simulink model "week14"  (R2018a)
settings: Solver=VariableStepAuto  StartTime=0.0  StopTime=15  RelTol=1e-3
values from neighbouring files (symbols this model uses):
  km = 0.5    [Parameters.m]    (also in Parameters.mat; parametersAcc.m; parametersPos.m; parametersVel.m)
  KP = 5    [Parameters.m]    (also in Parameters.mat; parametersAcc.m = 26; parametersPos.m; parametersVel.m)
  kTP = 1    [Parameters.m]    (also in Parameters.mat; parametersAcc.m; parametersPos.m; parametersVel.m)
  Tm = 0    [Parameters.m]    (also in Parameters.mat = 5; parametersAcc.m = 0.025; parametersPos.m = 0.025; parametersVel.m = 0.025)
  TP = 0    [Parameters.m]    (also in Parameters.mat = 5; parametersAcc.m = 2.5; parametersPos.m = 2.5; parametersVel.m = 2.5)
libraries: simulink x1
settings Model: Creator=Nguyen Mai  LastModifiedBy=Nguyen Mai

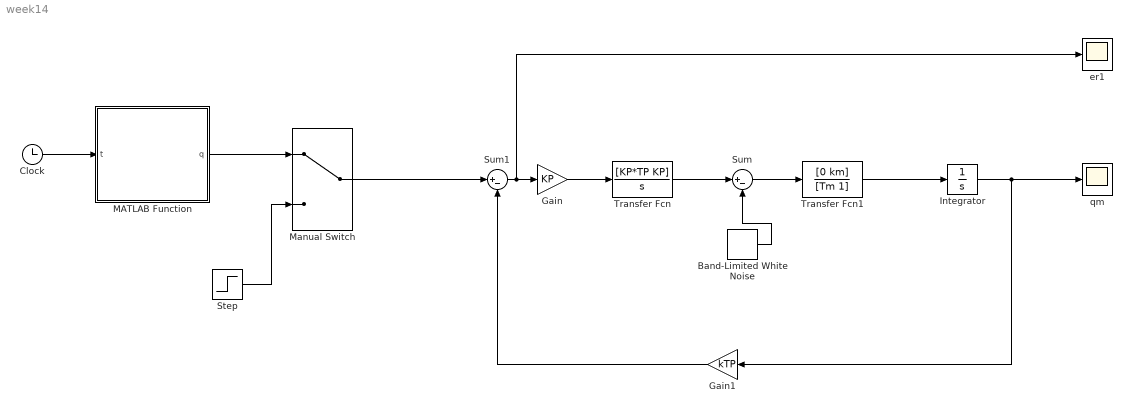
== system week14 ==
  Band-Limited White Noise : simulink/Sources/Band-Limited White Noise  Cov=[0.1]  Ts=0.1  seed=[23341]
  Clock : Clock
  Gain : Gain  Gain=KP
  Gain1 : Gain  Gain=kTP
  Integrator : Integrator
  MATLAB Function : MATLAB Function  TreatAsAtomicUnit=on
  Manual Switch : ManualSwitch
  Step : Step  SampleTime=0
  Sum : Sum  Inputs=|+-
  Sum1 : Sum  Inputs=|+-
  Transfer Fcn : TransferFcn  Numerator=[KP*TP KP]  Denominator=[1 0]
  Transfer Fcn1 : TransferFcn  Numerator=[0 km]  Denominator=[Tm 1]
  er1 : Scope
  qm : Scope
  wires:
  Sum1/1 -> er1/1, Gain/1
  Integrator/1 -> Gain1/1, qm/1
  Transfer Fcn/1 -> Sum/1
  Transfer Fcn1/1 -> Integrator/1
  Gain1/1 -> Sum1/2
  Band-Limited White Noise/1 -> Sum/2
  Sum/1 -> Transfer Fcn1/1
  Gain/1 -> Transfer Fcn/1
  Clock/1 -> MATLAB Function/1(t)
  MATLAB Function/1(q) -> Manual Switch/1
  Step/1 -> Manual Switch/2
  Manual Switch/1 -> Sum1/1

== matlab function week14/MATLAB Function ==
  data: t input; q output
function q = fcn(t)
t0=0;
tf=40;
tc=4/5;
if t<tc
q=40+(125/8)*t^2;
else
if t<tf-tc
q=30+25*t;
else
q=1020-(125/8)*(40-t)^2;
end
end
